simulink model "sensors"  (R2015b)
settings: Solver=ode1  StartTime=0.0  StopTime=Inf  FixedStep=0.001  RelTol=1e-3
PostLoadFcn:
  | , if any(exist('dsrtsu_mdlpostloadfcn', 'file') == [2, 3, 6]), try dsrtsu_mdlpostloadfcn('Execute', bdroot); catch fprintf('Error in PostLoadFcn (dsrtsu_mdlpostloadfcn) for model "%s":\n %s\n', bdroot, lasterr); end, end,
undefined symbols (not defined in the file or in its folder): canChannel
libraries: canlib x3, canmsglib x2, dspswit3 x1, powerlib_meascontrol x1, sldrtlib x1
settings Model: DSRTSU_INTERNAL_RTI_VER=460  DSRTSU_INTERNAL_RTI_TYPE=rti1401  DSRTSU_INTERNAL_RTIFPGA=50  Creator=luis  LastModifiedBy=luis
settings OptimizationCC: BlockReduction=off  OptimizeBlockIOStorage=off  BufferReuse=off  GlobalBufferReuse=off  ExpressionFolding=off  LocalBlockOutputs=off
settings HardwareCC: ProdEndianess=BigEndian  ProdWordSize=32  ProdHWDeviceType=Generic->Custom  TargetIntDivRoundTo=Zero  TargetEndianess=BigEndian  TargetHWDeviceType=Generic->Custom
settings RTWCC: SystemTargetFile=rti1401.tlc  MakeCommand=make_rti  TemplateMakefile=rti1401.tmf  Description=dSPACE DS1401 Hardware Platform
settings STFCustomTargetCC: ParMdlRefBuildCompliant=on  ConcurrentExecutionCompliant=off  GeneratePreprocessorConditionals=Use local settings  MatFileLogging=on  CPPClassGenCompliant=off  SystemTargetFile=rti1401.tlc
settings GRTTargetCC: CompOptLevelCompliant=off  ConcurrentExecutionCompliant=off  CombineOutputUpdateFcns=off  CPPClassGenCompliant=off  GRTInterface=on  UseToolchainInfoCompliant=off  ExtModeMexFile=noextcomm

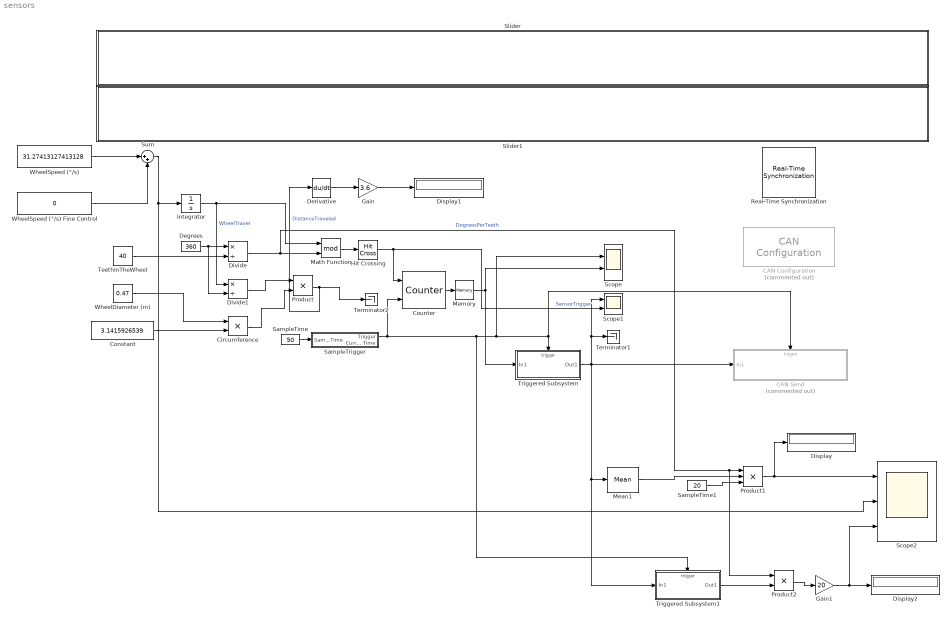
== system sensors ==
  CAN Configuration : canlib/CAN Configuration  Commented=on  BlockHandle=5.0001  DeviceMenu=(none)  Device=PEAK-System PCAN-USB (PCAN_USBBUS1)  ObjConstructor=canChannel('PEAK-System', 'PCAN_USBBUS1')  BusSpeed=500000  EnableBitParameters=off  SJW=NaN  TSEG1=NaN  TSEG2=NaN  NSamples=NaN  AckMode=Normal
  CAN Send : Subsystem  Commented=on
  Circumference : Product
  Constant : Constant  Value=3.1415926539
  Counter : dspswit3/Counter  Direction=Up  CountEvent=Rising edge  CounterSize=User defined  MaxCount=255  InitialCount=0  Output=Count  HitValue=32  ResetInput=on  SamplesPerFrame=1  Ts=1  CntDtype=double  HitDtype=Logical
  Degrees : Constant  Value=360
  Derivative : Derivative  CoefficientInTFapproximation=1
  Display : Display
  Display1 : Display
  Display2 : Display
  Divide : Product  Inputs=*/
  Divide1 : Product  Inputs=*/
  Gain : Gain  Gain=3.6
  Gain1 : Gain  Gain=20
  Hit Crossing : HitCross  HitCrossingOffset=6  HitCrossingDirection=falling
  Integrator : Integrator  WrappedStateUpperValue=360  WrappedStateLowerValue=0
  Math Function : Math  Operator=mod  SaturateOnIntegerOverflow=on
  Mean1 : powerlib_meascontrol/Measurements/Mean  Freq=5  Vinit=0  Ts=0
  Memory : Memory
  Product : Product
  Product1 : Product  Inputs=3
  Product2 : Product
  Real-Time Synchronization : sldrtlib/Real-Time Synchronization  SampleTime=0.001  MaxMissedTicks=100000000  ShowMissedTicks=off  YieldWhenWaiting=on
  SampleTime : Constant  Value=50
  SampleTime1 : Constant  Value=20
  SampleTrigger : Subsystem
  Scope : Scope  NumInputPorts=5
  Scope1 : Scope  NumInputPorts=2
  Scope2 : Scope  NumInputPorts=3
  Slider : Subsystem  DialogController=hmiCreateDDGDialog  IsWebBlock=on  mask(MWDashboardBlock){webBlockId=2ca2e308-2864-46cf-b624-a5bba4b8564e, webBlockType=slider, ShowInLibBrowser=on, ShowInitialText=on, HMISrcModelName=sensors}
      mask prompts: webBlockId "WebBlock Id"; webBlockType "WebBlock Type"; HMISrcModelName "Source Model"
      mask Help: helpview([docroot '/mapfiles/simulink.map'], 'hmi_slider')
      mask Display:
      | if strcmp(get_param(bdroot(gcb),'BlockDiagramType'), 'library')
      |     image([(matlabroot) '/toolbox/simulink/hmi/icons/Slider.png']);
      | end
  Slider1 : Subsystem  DialogController=hmiCreateDDGDialog  IsWebBlock=on  mask(MWDashboardBlock){webBlockId=df120065-c0d5-4740-9dfb-bba3dbed7d1d, webBlockType=slider, ShowInLibBrowser=on, ShowInitialText=on, HMISrcModelName=sensors}
      mask prompts: webBlockId "WebBlock Id"; webBlockType "WebBlock Type"; HMISrcModelName "Source Model"
      mask Help: helpview([docroot '/mapfiles/simulink.map'], 'hmi_slider')
      mask Display:
      | if strcmp(get_param(bdroot(gcb),'BlockDiagramType'), 'library')
      |     image([(matlabroot) '/toolbox/simulink/hmi/icons/Slider.png']);
      | end
  Sum : Sum  Inputs=|++
  TeethInTheWheel : Constant  Value=40
  Terminator1 : Terminator
  Terminator2 : Terminator
  Triggered Subsystem : Subsystem  TreatAsAtomicUnit=on
  Triggered Subsystem1 : Subsystem  TreatAsAtomicUnit=on
  WheelDiameter (m) : Constant  Value=0.47
  WheelSpeed (°/s) : Constant  Value=31.27413127413128
  WheelSpeed (°/s) Fine Control : Constant  Value=0
  wires:
  Integrator/1 -> Divide1/1, Math Function/1  "WheelTravel"
  Degrees/1 -> Divide1/2, Divide/1
  TeethInTheWheel/1 -> Divide/2
  Divide/1 -> Product2/1, Product1/1, Math Function/2  "DegreesPerTeeth"
  Hit Crossing/1 -> Counter/1, Scope1/2  "SensorTrigger"
  Math Function/1 -> Hit Crossing/1
  SampleTime/1 -> SampleTrigger/1(SampleTime)
  SampleTrigger/1(Trigger) -> Triggered Subsystem1/Trigger, Scope/2, Triggered Subsystem/Trigger, CAN Send/Trigger, Counter/2
  Memory/1 -> Scope/4, Triggered Subsystem/1(In1)
  Counter/1 -> Memory/1
  WheelDiameter (m)/1 -> Circumference/1
  Constant/1 -> Circumference/2
  Divide1/1 -> Product/1
  Circumference/1 -> Product/2
  Product/1 -> Derivative/1, Terminator2/1  "DistanceTraveled"
  Mean1/1 -> Product1/2
  SampleTime1/1 -> Product1/3
  Product1/1 -> Display/1, Scope2/1
  Derivative/1 -> Gain/1
  Gain/1 -> Display1/1
  Triggered Subsystem/1(Out1) -> CAN Send/1(In1), Triggered Subsystem1/1(In1), Mean1/1, Terminator1/1, Scope1/1
  Triggered Subsystem1/1(Out1) -> Product2/2
  Product2/1 -> Gain1/1
  Gain1/1 -> Display2/1, Scope2/3
  Sum/1 -> Scope2/2, Integrator/1
  WheelSpeed (°/s)/1 -> Sum/1
  WheelSpeed (°/s) Fine Control/1 -> Sum/2

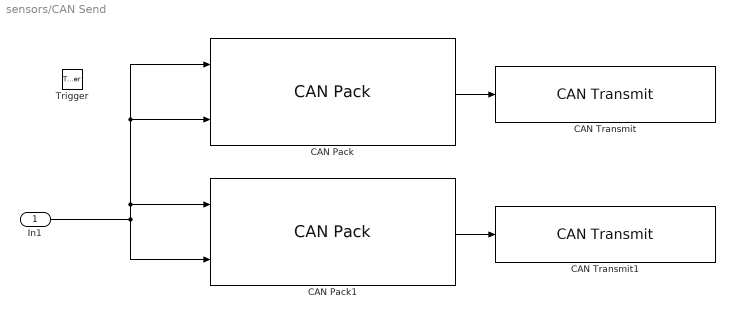
== system sensors/CAN Send ==
  In1 : Inport
  Trigger : TriggerPort  PortDimensions=1
  CAN Pack : canmsglib/CAN Pack  CANdbFile=C:\Users\luis\Documents\tuc racing\mainECU\database\main_0_4.dbc  MsgList=ciBox_Front_PDO1  MsgName=ciBox_Front_PDO1  MsgIDType=Standard (11-bit identifier)  MsgIdentifier=386  MsgLength=8  SignalInfo=Wheel_Speed_Front_Left$0$16$1$2$1$0$1$0$-Inf$Inf$#Wheel_Speed_Front_Right$16$16$1$2$1$0$1$0$-Inf$Inf$#  NSignals=2  StartBits=str2num('[int32(0);int32(16)]')  SignalSizes=str2num('[int32(16);int32(16)]')  ByteOrders=str2num('[int32(1);int32(1)]')  DataTypes=str2num('[int32(2);int32(2)]')  MultiplexTypes=str2num('[int32(1);int32(1)]')  MultiplexValues=str2num('[double(0);double(0)]')  Factors=str2num('[double(1);double(1)]')  Offsets=str2num('[double(0);double(0)]')  Minimums=str2num('[double(-Inf);double(-Inf)]')  Maximums=str2num('[double(Inf);double(Inf)]')  Remote=off
      settings: DataFormat=CANdb specified signals
  CAN Pack1 : canmsglib/CAN Pack  CANdbFile=C:\Users\luis\Documents\tuc racing\mainECU\database\main_0_4.dbc  MsgList=ciBox_Rear_PDO1  MsgName=ciBox_Rear_PDO1  MsgIDType=Standard (11-bit identifier)  MsgIdentifier=392  MsgLength=8  SignalInfo=Wheel_Speed_Rear_Left$0$16$1$2$1$0$1$0$-Inf$Inf$#Wheel_Speed_Rear_Right$16$16$1$2$1$0$1$0$-Inf$Inf$#  NSignals=2  StartBits=str2num('[int32(0);int32(16)]')  SignalSizes=str2num('[int32(16);int32(16)]')  ByteOrders=str2num('[int32(1);int32(1)]')  DataTypes=str2num('[int32(2);int32(2)]')  MultiplexTypes=str2num('[int32(1);int32(1)]')  MultiplexValues=str2num('[double(0);double(0)]')  Factors=str2num('[double(1);double(1)]')  Offsets=str2num('[double(0);double(0)]')  Minimums=str2num('[double(-Inf);double(-Inf)]')  Maximums=str2num('[double(Inf);double(Inf)]')  Remote=off
      settings: DataFormat=CANdb specified signals
  CAN Transmit : canlib/CAN Transmit  BlockHandle=11.0002  DeviceMenu=(none)  Device=PEAK-System PCAN-USB (PCAN_USBBUS1)  ObjConstructor=canChannel('PEAK-System', 'PCAN_USBBUS1')  EnablePeriodicTransmit=off  MessagePeriod=0
  CAN Transmit1 : canlib/CAN Transmit  BlockHandle=12.0002  DeviceMenu=(none)  Device=PEAK-System PCAN-USB (PCAN_USBBUS1)  ObjConstructor=canChannel('PEAK-System', 'PCAN_USBBUS1')  EnablePeriodicTransmit=off  MessagePeriod=0
  wires:
  CAN Pack/1 -> CAN Transmit/1
  CAN Pack1/1 -> CAN Transmit1/1
  In1/1 -> CAN Pack/1, CAN Pack/2, CAN Pack1/1, CAN Pack1/2

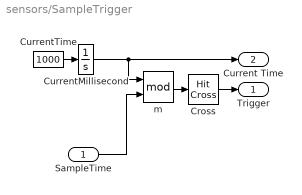
== system sensors/SampleTrigger ==
  SampleTime : Inport
  Cross : HitCross  HitCrossingOffset=1  HitCrossingDirection=falling
  CurrentMillisecond : Integrator  WrappedStateUpperValue=360  WrappedStateLowerValue=0
  CurrentTime : Constant  Value=1000
  m : Math  Operator=mod  SaturateOnIntegerOverflow=on
  Trigger : Outport
  Current Time : Outport  Port=2
  wires:
  m/1 -> Cross/1
  CurrentMillisecond/1 -> Current Time/1, m/1
  SampleTime/1 -> m/2
  Cross/1 -> Trigger/1
  CurrentTime/1 -> CurrentMillisecond/1

== system sensors/Slider ==

== system sensors/Slider1 ==

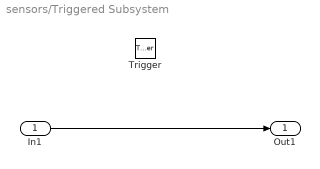
== system sensors/Triggered Subsystem ==
  In1 : Inport
  Trigger : TriggerPort
  Out1 : Outport
  wires:
  In1/1 -> Out1/1

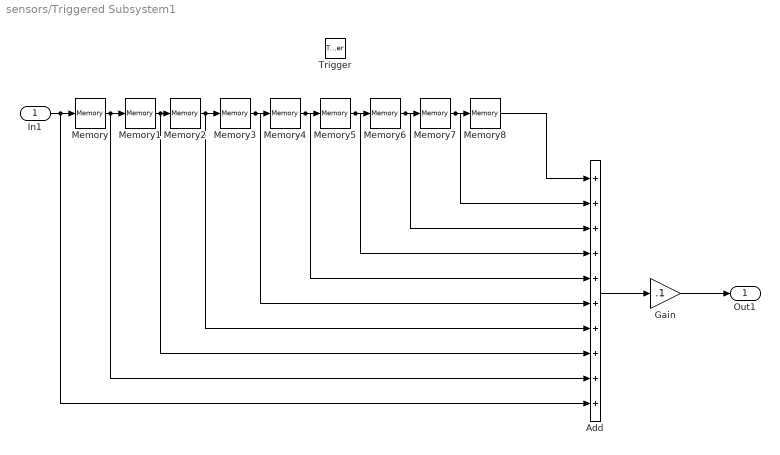
== system sensors/Triggered Subsystem1 ==
  In1 : Inport
  Trigger : TriggerPort
  Add : Sum  Inputs=++++++++++
  Gain : Gain  Gain=.1
  Memory{,1..8} (9 alike) : Memory  InheritSampleTime=on
  Out1 : Outport
  wires:
  Memory/1 -> Add/9, Memory1/1
  Memory1/1 -> Add/8, Memory2/1
  Memory3/1 -> Add/6, Memory4/1
  Memory4/1 -> Add/5, Memory5/1
  Memory5/1 -> Add/4, Memory6/1
  Memory6/1 -> Add/3, Memory7/1
  Memory7/1 -> Add/2, Memory8/1
  In1/1 -> Add/10, Memory/1
  Memory2/1 -> Add/7, Memory3/1
  Add/1 -> Gain/1
  Gain/1 -> Out1/1
  Memory8/1 -> Add/1
